simulink model "index"  (R2024b)
settings: Solver=FixedStepAuto  StartTime=0.0  StopTime=1000.0  FixedStep=0.001  RelTol=1e-3
libraries: config x1, notificaStato x1, luci x1, rgbled_temp x1
settings Model: Creator=mainuser  LastModifiedBy=mainuser

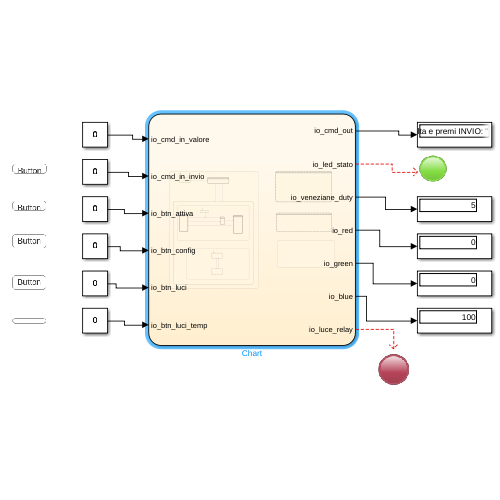
[thumbnail: Simulink's stored preview of the top-level diagram]
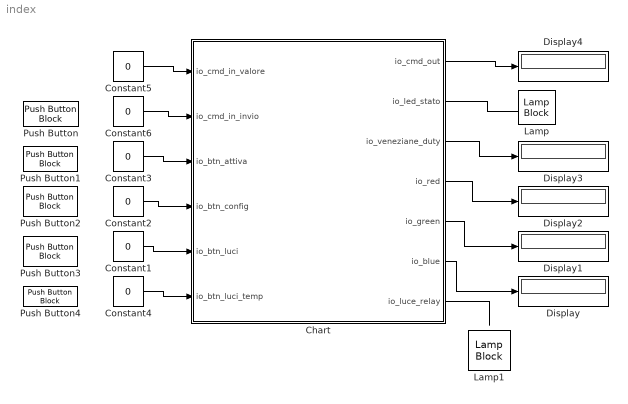
== system index ==
  Chart : Stateflow chart  TreatAsAtomicUnit=on
  Constant{1..4,6} (5 alike) : Constant  Value=0  OutDataTypeStr=boolean
  Constant5 : Constant  Value=0  OutDataTypeStr=uint8
  Display{,1..4} (5 alike) : Display
  Lamp : LampBlock  LabelPosition=Hide
  Lamp1 : LampBlock  LabelPosition=Hide
  Push Button{,1,3..4} (4 alike) : PushButtonBlock  OffValue=0.000000
  Push Button2 : PushButtonBlock
  wires:
  Constant6/1 -> Chart/2(io_cmd_in_invio)
  Constant3/1 -> Chart/3(io_btn_attiva)
  Constant2/1 -> Chart/4(io_btn_config)
  Constant1/1 -> Chart/5(io_btn_luci)
  Constant4/1 -> Chart/6(io_btn_luci_temp)
  Constant5/1 -> Chart/1(io_cmd_in_valore)
  Chart/6(io_blue) -> Display/1
  Chart/5(io_green) -> Display1/1
  Chart/4(io_red) -> Display2/1
  Chart/3(io_veneziane_duty) -> Display3/1
  Chart/1(io_cmd_out) -> Display4/1
  Chart/2(io_led_stato) -> ?
  Chart/7(io_luce_relay) -> ?

== stateflow chart index/Chart ==
  state Attivita [parallel]
    settings: executionOrder=1
    state Inattivo
      en:
      io_led_stato=false
      config_veneziane_gradi=0
      config_luci_sec=0
      config_temp_rgb=16
    state Start
      config_is_valida=false
    state Atttivo
      state Attivo_Interfaccia [parallel]
        settings: executionOrder=1
        state Attivo_start
        state Config
        state NotificaStato
        state AttivaNewconf
          config_veneziane_gradi=newconfig_veneziane_gradi
          config_luci_sec=newconfig_veneziane_gradi
          config_temp_rgb=newconfig_temp_rgb
        (default) -> Attivo_start
        Attivo_start -> (junction 89)
        (junction 89) -> AttivaNewconf [order 2]
        (junction 89) -> Config [order 1] : [config_is_valida==false]
        AttivaNewconf -> NotificaStato
        145 -> AttivaNewconf : {config_is_valida=true}
        NotificaStato -> Config : [hasChangedTo(io_btn_config,true)]
      state Attivita_LED [parallel]
        settings: executionOrder=2
        state Attivo_ON
          en: io_led_stato=true;
        state Attivo_OFF
          en: io_led_stato=false;
        (default) -> Attivo_ON
        Attivo_ON -> Attivo_OFF : after(0.5,sec)
        Attivo_OFF -> Attivo_ON : after(0.5,sec)
    (default) -> Start
    Start -> Inattivo
    Atttivo -> Inattivo : [hasChangedTo(io_btn_attiva,true)]
    Inattivo -> Atttivo : [hasChangedTo(io_btn_attiva,true)]
  state Luci [parallel]
    settings: executionOrder=2
  state RGBLED_TEMP [parallel]
    settings: executionOrder=4
  state Veneziane [parallel]
    io_veneziane_duty = (config_veneziane_gradi / 180) * 5 + 5;
    settings: executionOrder=3
  data: config_veneziane_gradi function_output; config_luci_sec function_output; config_temp function_output; config_luci_stato function_output; state_temp function_input; state_veneziane_gradi function_input; state_stato_luce function_input; config_temp_sec function_input; config_luce_state function_input; io_temp function_input; config_is_valida local boolean size=1; io_cmd_out output string; io_cmd_in_valore input uint8; io_cmd_in_invio input; newconfig_veneziane_gradi local uint8 size=1; config_veneziane_gradi local uint8 size=1; newconfig_luci_sec local uint8 size=1; config_luci_sec local uint8 size=1; newconfig_temp_rgb local uint8 size=1; config_temp_rgb local uint8 size=1; io_btn_attiva input boolean size=1; io_btn_config input boolean size=1; io_led_stato output boolean size=1; io_btn_luci input boolean size=1; io_btn_luci_temp input boolean size=1; config_luci_state local boolean size=1; io_luce_stato local boolean size=1; io_veneziane_duty output; io_red output double size=1; io_green output double size=1; io_blue output double size=1; io_luce_relay output boolean size=1
